simulink model "tepeRarx"  (R2019a)
settings: Solver=VariableStepAuto  StartTime=0.0  StopTime=3  FixedStep=Ts_Power  RelTol=1e-4
PreLoadFcn:
  | Ts_Power=50e-6;
  | Slope_Vdc=1;
InitFcn:
  | Ts_Power=50e-6;
  | Tc=1e-5;%break algebraic loop time constant
  | BlockName=[gcs,'/m11'];
  | ModuleName=get_param(BlockName,'ModuleName');
  | Voc1=str2num(get_param(BlockName,'Voc'));
  | Nser1=str2num(get_param(BlockName,'Nser'));
  | Slope_Vdc=Nser1*Voc1;
StopFcn:
  | if exist('I','var') && exist('V','var')
  |    figure(1)
  |    clf
  |    n=find(Itot>=0);
  |    n=n(end);
  |    Vglobal=Vtot(1:n);
  |    Iglobal=Itot(1:n);
  | 
  | 
  |    Pglobal=Vglobal.*Iglobal;
  |    n=find(Pglobal==max(Pglobal));
  |    Pmax=Pglobal(n);
  |    Vmp=Vglobal(n);
  |    Imp=Iglobal(n);
  | 
  | 
  |    subplot(211)
  |    plot(Vglobal, Iglobal,Vmp,Imp,'or')
  |    ylabel('Current (A)')
  |    title(sprintf('Global I-V & P-V characteristics\n %s' ,ModuleName))
  | 
  | 
  |    subplot(212)
  |    plot(Vglobal, Pglobal,Vmp,Pmax,'or')
  |    ylabel('Power (W)')
  |    xlabel('Voltage (V)')
  | end
undefined symbols (not defined in the file or in its folder): Irr
libraries: powerlib x16, re_lib x9, simulink x1
Description:
  | Copyright 2008-2019 The MathWorks, Inc.
settings Model: Creator=MathWorks  LastModifiedBy=makis
settings SolverCC: AlgebraicLoopSolver=LineSearch
settings DataIOCC: LimitDataPoints=on  SaveFormat=Array  SignalLoggingSaveFormat=ModelDataLogs  ReturnWorkspaceOutputs=off
settings OptimizationCC: ExpressionDepthLimit=2147483647  LifeSpan=inf
settings DebuggingCC: UnderspecifiedInitializationDetection=Classic  MergeDetectMultiDrivingBlocksExec=none  SolverPrmCheckMsg=warning  FcnCallInpInsideContextMsg=warning  AllowSymbolicDim=off  StateNameClashWarn=warning  SFUnexpectedBacktrackingDiag=warning  SFNoUnconditionalDefaultTransitionDiag=warning  SFExecutionAtInitializationDiag=none  ArithmeticOperatorsInVariantConditions=warning
settings HardwareCC: ProdBitPerPointer=32  ProdBitPerSizeT=32  ProdBitPerPtrDiffT=32  ProdLargestAtomicFloat=None  ProdIntDivRoundTo=Undefined  ProdEndianess=Unspecified  ProdWordSize=32  ProdHWDeviceType=32-bit Generic
settings ModelReferenceCC: PropagateSignalLabelsOutOfModel=off
settings SFSimCC: SimUseLocalCustomCode=off
settings RTWCC: RTWUseLocalCustomCode=off
settings CodeAppCC: StateflowObjectComments=on
settings GRTTargetCC: TargetLangStandard=C89/C90 (ANSI)  GeneratePreprocessorConditionals=Disable all  CombineOutputUpdateFcns=off  GRTInterface=on
settings ConfigComp: CovMetricSettings=dw  CovHtmlReporting=on  CovSaveCumulativeToWorkspaceVar=on  CovSaveSingleToWorkspaceVar=on  CovExternalEMLEnable=off  CovSFcnEnable=off
settings SimscapeCC: SimscapeNormalizeSystem=off

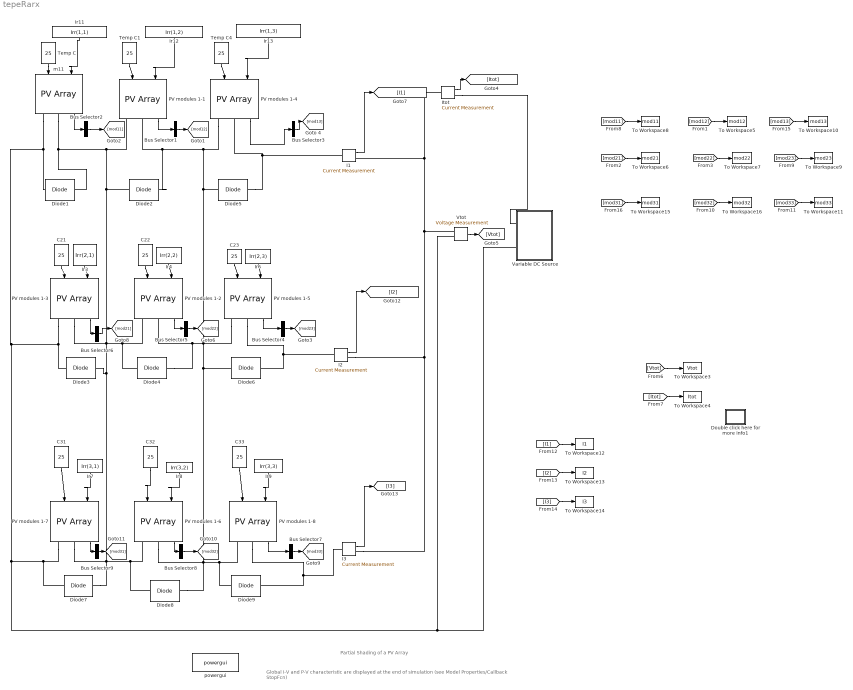
== system tepeRarx ==
  note: Global I-V and P-V characteristic are displayed at the end of simulation
      | (see Model Properties/Callback StopFcn)
  note: Partial Shading of a PV Array
  Bus Selector{1..9} (9 alike) : BusSelector  OutputSignals=V_PV,I_PV  OutputAsBus=on
  C{21..23,31..33} (6 alike) : Constant  Value=25
  Diode{1..9} (9 alike) : powerlib/Power Electronics/Diode  Ron=0.001  Lon=0  Vf=0.7  IC=0  UseSnubber=off  Rs=1e5*inf  Cs=inf  Measurements=off
      settings: SourceProductName=Simscape Electrical
  Double click here for more info1 : Subsystem
      settings: OpenFcn=showdemo(bdroot(gcb))
      mask Display: disp('?')
  I1 : powerlib/Measurements/Current Measurement  PhasorSimulation=off  OutputType=Complex  PSBequivalent=0
      settings: SourceProductName=Simscape Electrical
  I2 : powerlib/Measurements/Current Measurement  PhasorSimulation=off  OutputType=Complex  PSBequivalent=0
      settings: SourceProductName=Simscape Electrical
  I3 : powerlib/Measurements/Current Measurement  PhasorSimulation=off  OutputType=Complex  PSBequivalent=0
      settings: SourceProductName=Simscape Electrical
  "Ir11 " : Constant  Value=Irr(1,1)  VectorParams1D=off
  "Ir12 " : Constant  Value=Irr(1,2)  VectorParams1D=off
  Ir13 : Constant  Value=Irr(1,3)  VectorParams1D=off
  Ir3 : Constant  Value=Irr(2,1)
  Ir4 : Constant  Value=Irr(2,2)
  Ir6 : Constant  Value=Irr(2,3)
  Ir7 : Constant  Value=Irr(3,1)
  Ir8 : Constant  Value=Irr(3,2)
  Ir9 : Constant  Value=Irr(3,3)
  Itot : powerlib/Measurements/Current Measurement  PhasorSimulation=off  OutputType=Complex  PSBequivalent=0
      settings: SourceProductName=Simscape Electrical
  PV modules 1-{1..8} (8 alike) : re_lib/Solar/PV Array  Npar=1  Nser=1  PlotType=array @ 25 deg.C & specified irradiances  S_vec="[ 1000  500  100 ]"  Temp_C_vec="[ 45 25  ]"  ModuleName=User-defined  PlotWhenSelected=off  Pm=83.2824  Ncell=60/3  Voc=37.92*20/60  Isc=8.62  Vm=30.96*20/60  Im=8.07  beta_Voc_pc=-0.33969  alpha_Isc_pc=0.063701  beta_Voc=-0.042937  alpha_Isc=0.005491  IL=8.6307  I0=1.4176e-10  nI=0.99132  Rsh=82.1161  Rs=0.098625  BAL=on  Tc=Tc  Tfilter=5e-5
      settings: SourceProductName=Simscape Electrical
  Temp C : Constant  Value=25
  Temp C1 : Constant  Value=25
  Temp C4 : Constant  Value=25
  To Workspace10 : ToWorkspace  VariableName=mod13  SampleTime=1e-3
  To Workspace11 : ToWorkspace  VariableName=mod33  SampleTime=1e-3
  To Workspace12 : ToWorkspace  VariableName=I1  SampleTime=1e-3
  To Workspace13 : ToWorkspace  VariableName=I2  SampleTime=1e-3
  To Workspace14 : ToWorkspace  VariableName=I3  SampleTime=1e-3
  To Workspace15 : ToWorkspace  VariableName=mod31  SampleTime=1e-3
  To Workspace16 : ToWorkspace  VariableName=mod32  SampleTime=1e-3
  To Workspace3 : ToWorkspace  VariableName=Vtot  SampleTime=1e-3
  To Workspace4 : ToWorkspace  VariableName=Itot  SampleTime=1e-3
  To Workspace5 : ToWorkspace  VariableName=mod12  SampleTime=1e-3
  To Workspace6 : ToWorkspace  VariableName=mod21  SampleTime=1e-3
  To Workspace7 : ToWorkspace  VariableName=mod22  SampleTime=1e-3
  To Workspace8 : ToWorkspace  VariableName=mod11  SampleTime=1e-3
  To Workspace9 : ToWorkspace  VariableName=mod23  SampleTime=1e-3
  Variable DC Source : Subsystem
  Vtot : powerlib/Measurements/Voltage Measurement  PhasorSimulation=off  OutputType=Complex  PSBequivalent=0
      settings: SourceProductName=Simscape Electrical
  m11 : re_lib/Solar/PV Array  Npar=1  Nser=1  PlotType=array @ 25 deg.C & specified irradiances  S_vec="[ 1000  500  100 ]"  Temp_C_vec="[ 45 25  ]"  ModuleName=User-defined  PlotWhenSelected=off  Pm=83.2824  Ncell=60/3  Voc=37.92*20/60  Isc=8.62  Vm=30.96*20/60  Im=8.07  beta_Voc_pc=-0.33969  alpha_Isc_pc=0.063701  beta_Voc=-0.042937  alpha_Isc=0.005491  IL=8.6307  I0=1.4176e-10  nI=0.99132  Rsh=82.1161  Rs=0.098625  BAL=on  Tc=Tc  Tfilter=5e-5
      settings: SourceProductName=Simscape Electrical
  powergui : powerlib/powergui  Priority=1  SimulationMode=Continuous  SampleTime=Ts_Power*0 + 20e-6  frequency=60  Iterations=50  frequencyindice=0  Pbase=100e6  ErrMax=1e-4  UnitsV=kV  UnitsW=MW  buscounter=0  FunctionMessages=off  echomessages=off  EnableUseOfTLC=off  CurrentSourceSwitches=on  DisableSnubberDevices=on  DisableRonSwitches=off  DisableVfSwitches=off  DisplayEquations=off  AutomaticDiscreteSolvers=off  SolverType=Tustin/Backward Euler (TBE)  Interpol=off  ExternalGateDelay=off  methode=off  Ts=0  x0status=blocks  SPID=off  SwTol=0  HookPort=off  NonlinearTolerance=0  nMaxIteration=15  ContinueOnMaxIteration=off  RestoreLinks=warning  ResistiveCurrentMeasurement=off  Frange=[0:2:500]  Ylog=off  Xlog=on  ShowGrid=off  save=off  variable=ZData  structure=0  ZoomFFT=on  StartTime=0.0  cycles=1  DisplayStyle=1  fundamental=60  FreqAxis=off  MaxFrequency=1000  frequencyindicesteady=1  RmsSteady=1  display=off
      settings: SourceProductName=Simscape Electrical
  wires:
  PV modules 1-7/1 -> Bus Selector9/1
  Bus Selector6/1 -> [mod21]
  I3/1 -> [I3]
  PV modules 1-3/1 -> Bus Selector6/1
  I1/1 -> [I1]
  [I1] -> To Workspace12/1
  [mod22] -> To Workspace7/1
  I2/1 -> [I2]
  Ir9/1 -> PV modules 1-8/1
  Bus Selector5/1 -> [mod22]
  [I3] -> To Workspace14/1
  Bus Selector9/1 -> [mod31]
  [I2] -> To Workspace13/1
  Temp C1/1 -> PV modules 1-1/2
  Bus Selector8/1 -> [mod32]
  [mod33] -> To Workspace11/1
  Ir4/1 -> PV modules 1-2/1
  PV modules 1-5/1 -> Bus Selector4/1
  Bus Selector4/1 -> [mod23]
  Ir6/1 -> PV modules 1-5/1
  m11/1 -> Bus Selector2/1
  PV modules 1-2/1 -> Bus Selector5/1
  [mod32] -> To Workspace16/1
  [mod31] -> To Workspace15/1
  Itot/1 -> [Itot]
  [mod23] -> To Workspace9/1
  [mod21] -> To Workspace6/1
  PV modules 1-6/1 -> Bus Selector8/1
  Bus Selector7/1 -> [mod33]
  PV modules 1-4/1 -> Bus Selector3/1
  Ir3/1 -> PV modules 1-3/1
  PV modules 1-8/1 -> Bus Selector7/1
  [mod11] -> To Workspace8/1
  [mod12] -> To Workspace5/1
  Bus Selector2/1 -> [mod11]
  Bus Selector1/1 -> [mod12]
  PV modules 1-1/1 -> Bus Selector1/1
  [mod13] -> To Workspace10/1
  Bus Selector3/1 -> [mod13]
  "Ir12 "/1 -> PV modules 1-1/1
  Ir13/1 -> PV modules 1-4/1
  C22/1 -> PV modules 1-2/2
  "Ir11 "/1 -> m11/1
  C33/1 -> PV modules 1-8/2
  C32/1 -> PV modules 1-6/2
  Ir8/1 -> PV modules 1-6/1
  C31/1 -> PV modules 1-7/2
  Ir7/1 -> PV modules 1-7/1
  C23/1 -> PV modules 1-5/2
  C21/1 -> PV modules 1-3/2
  Vtot/1 -> [Vtot]
  [Itot] -> To Workspace4/1
  [Vtot] -> To Workspace3/1
  Temp C/1 -> m11/2
  Temp C4/1 -> PV modules 1-4/2
  connections:
  Diode6/RConn1 -- PV modules 1-5/RConn1 -- I2/LConn1
  I2/RConn1 -- Vtot/LConn1 -- I1/RConn1 -- Itot/LConn1 -- I3/RConn1
  Diode9/RConn1 -- PV modules 1-8/RConn1 -- I3/LConn1
  Variable DC Source/LConn2 -- Vtot/LConn2 -- m11/RConn2 -- Diode1/LConn1 -- Diode3/LConn1 -- PV modules 1-3/RConn2 -- Diode7/LConn1 -- PV modules 1-7/RConn2
  PV modules 1-1/RConn2 -- Diode1/RConn1 -- m11/RConn1 -- Diode2/LConn1 -- PV modules 1-3/RConn1 -- Diode4/LConn1 -- PV modules 1-2/RConn2 -- PV modules 1-7/RConn1 -- Diode7/RConn1 -- Diode8/LConn1 -- PV modules 1-6/RConn2 -- Diode3/RConn1
  PV modules 1-1/RConn1 -- Diode2/RConn1 -- PV modules 1-6/RConn1 -- Diode8/RConn1 -- PV modules 1-8/RConn2 -- Diode9/LConn1 -- Diode6/LConn1 -- Diode4/RConn1 -- PV modules 1-2/RConn1 -- PV modules 1-5/RConn2 -- Diode5/LConn1 -- PV modules 1-4/RConn2
  PV modules 1-4/RConn1 -- Diode5/RConn1 -- I1/LConn1
  Itot/RConn1 -- Variable DC Source/LConn1

== system tepeRarx/Double click here for more info1 ==

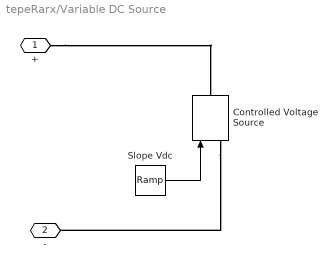
== system tepeRarx/Variable DC Source ==
  Controlled Voltage Source : powerlib/Electrical Sources/Controlled Voltage Source  Initialize=on  Source_Type=AC  Amplitude=0  Phase=0  Frequency=0  Measurements=None
      settings: SourceProductName=Simscape Electrical
  Slope Vdc : simulink/Sources/Ramp  slope=Slope_Vdc  start=0  InitialOutput=0
  + : PMIOPort  Side=Left
  - : PMIOPort  Port=2  Side=Left
  wires:
  Slope Vdc/1 -> Controlled Voltage Source/1
  connections:
  Controlled Voltage Source/LConn1 -- -/RConn1
  +/RConn1 -- Controlled Voltage Source/RConn1
